simulink model "posture_reg_with_odoloc_Euler"  (Simulink 8.7)
settings: Solver=ode45  StartTime=0.0  StopTime=T  MaxStep=0.01  RelTol=1e-3
values from neighbouring files (symbols this model uses):
  T_s = 0.01    [init.m]
  theta_0 = pi/2    (= 1.57079632679)    [init.m]
  x_0 = -1    [init.m]
  y_0 = -2    [init.m]
undefined symbols (not defined in the file or in its folder): post_reg, wrap
settings Model: Creator=marilena  LastModifiedBy=giuseppe  ExtModeAutoUpdateStatusClock=off
settings DataIOCC: SignalLoggingSaveFormat=ModelDataLogs
settings OptimizationCC: ExpressionDepthLimit=2147483647
settings DebuggingCC: SaveWithParameterizedLinksMsg=none  SolverPrmCheckMsg=warning  FcnCallInpInsideContextMsg=UseLocalSettings  StateNameClashWarn=warning
settings HardwareCC: TargetHWDeviceType=32-bit Generic
settings GRTTargetCC: TargetFcnLib=ansi_tfl_tmw.mat  GeneratePreprocessorConditionals=Use local settings  CombineOutputUpdateFcns=off  GRTInterface=on

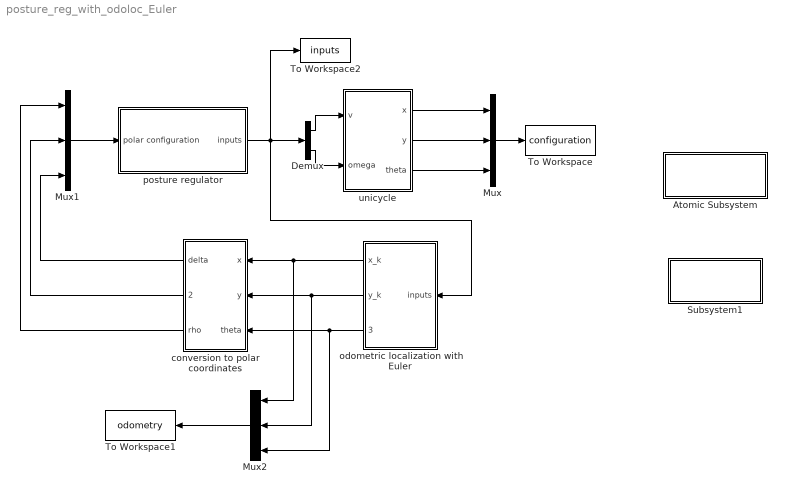
== system posture_reg_with_odoloc_Euler ==
  Atomic Subsystem : Subsystem  TreatAsAtomicUnit=on
      settings: OpenFcn=init
      mask Display: disp('initialization')
  Demux : Demux  Outputs=2
  Mux : Mux  Inputs=3
  Mux1 : Mux  Inputs=3
  Mux2 : Mux  Inputs=3
  Subsystem1 : Subsystem
      settings: OpenFcn=plots
      mask Display: disp('plots')
  To Workspace : ToWorkspace  VariableName=configuration  SaveFormat=Structure With Time
  To Workspace1 : ToWorkspace  VariableName=odometry  SaveFormat=Structure With Time
  To Workspace2 : ToWorkspace  VariableName=inputs  SaveFormat=Structure With Time
  conversion to polar coordinates : Subsystem
  odometric localization with Euler : Subsystem
  posture regulator : Subsystem
  unicycle : Subsystem
  wires:
  Mux/1 -> To Workspace/1
  unicycle/3(theta) -> Mux/3
  unicycle/1(x) -> Mux/1
  Mux1/1 -> posture regulator/1(polar configuration)
  posture regulator/1(inputs) -> odometric localization with Euler/1(inputs), Demux/1, To Workspace2/1
  unicycle/2(y) -> Mux/2
  Demux/1 -> unicycle/1(v)
  Demux/2 -> unicycle/2(omega)
  odometric localization with Euler/1(x_k) -> Mux2/1, conversion to polar coordinates/1(x)
  odometric localization with Euler/2(y_k) -> Mux2/2, conversion to polar coordinates/2(y)
  odometric localization with Euler/3(theta_k) -> Mux2/3, conversion to polar coordinates/3(theta)
  conversion to polar coordinates/1(delta) -> Mux1/3
  conversion to polar coordinates/2(gamma) -> Mux1/2
  conversion to polar coordinates/3(rho) -> Mux1/1
  Mux2/1 -> To Workspace1/1

== system posture_reg_with_odoloc_Euler/Atomic Subsystem ==

== system posture_reg_with_odoloc_Euler/Subsystem1 ==

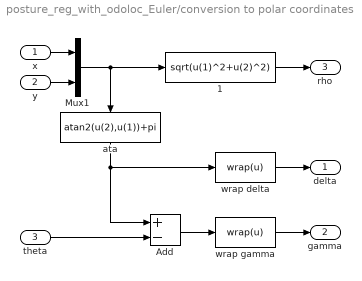
== system posture_reg_with_odoloc_Euler/conversion to polar coordinates ==
  x : Inport
  y : Inport  Port=2
  theta : Inport  Port=3
  " 1" : Fcn  Expr=sqrt(u(1)^2+u(2)^2)
  Add : Sum  Inputs=+-
  Mux1 : Mux  Inputs=2
  ata : Fcn  Expr=atan2(u(2),u(1))+pi
  wrap delta : MATLABFcn  MATLABFcn=wrap(u)
  wrap gamma : MATLABFcn  MATLABFcn=wrap(u)
  delta : Outport
  gamma : Outport  Port=2
  rho : Outport  Port=3
  wires:
  Mux1/1 -> " 1"/1, ata/1
  ata/1 -> Add/1, wrap delta/1
  x/1 -> Mux1/1
  " 1"/1 -> rho/1
  y/1 -> Mux1/2
  theta/1 -> Add/2
  wrap delta/1 -> delta/1
  Add/1 -> wrap gamma/1
  wrap gamma/1 -> gamma/1

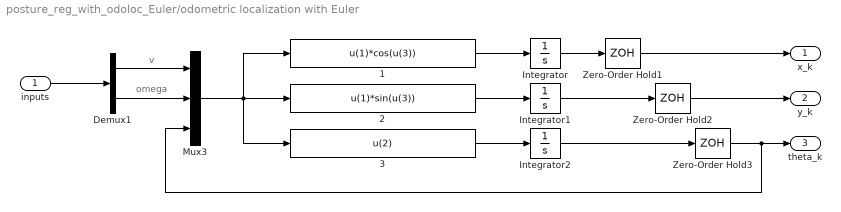
== system posture_reg_with_odoloc_Euler/odometric localization with Euler ==
  note: omega
  note: v
  inputs : Inport
  " 1" : Fcn  Expr=u(1)*cos(u(3))
  " 2" : Fcn  Expr=u(1)*sin(u(3))
  " 3" : Fcn  Expr=u(2)
  Demux1 : Demux  Outputs=2
  Integrator : Integrator  InitialCondition=x_0
  Integrator1 : Integrator  InitialCondition=y_0
  Integrator2 : Integrator  InitialCondition=theta_0
  Mux3 : Mux  Inputs=3
  Zero-Order Hold1 : ZeroOrderHold  SampleTime=T_s
  Zero-Order Hold2 : ZeroOrderHold  SampleTime=T_s
  Zero-Order Hold3 : ZeroOrderHold  SampleTime=T_s
  x_k : Outport
  y_k : Outport  Port=2
  theta_k : Outport  Port=3
  wires:
  " 1"/1 -> Integrator/1
  " 2"/1 -> Integrator1/1
  Mux3/1 -> " 3"/1, " 1"/1, " 2"/1
  " 3"/1 -> Integrator2/1
  Integrator/1 -> Zero-Order Hold1/1
  Integrator1/1 -> Zero-Order Hold2/1
  Integrator2/1 -> Zero-Order Hold3/1
  Zero-Order Hold3/1 -> Mux3/3, theta_k/1
  Zero-Order Hold2/1 -> y_k/1
  Zero-Order Hold1/1 -> x_k/1
  Demux1/1 -> Mux3/1
  Demux1/2 -> Mux3/2
  inputs/1 -> Demux1/1

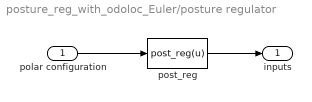
== system posture_reg_with_odoloc_Euler/posture regulator ==
  polar configuration : Inport
  post_reg : MATLABFcn  Tag={'prova'}  Description=cartesian regulator  MATLABFcn=post_reg(u)  Output1D=off
  inputs : Outport
  wires:
  polar configuration/1 -> post_reg/1
  post_reg/1 -> inputs/1

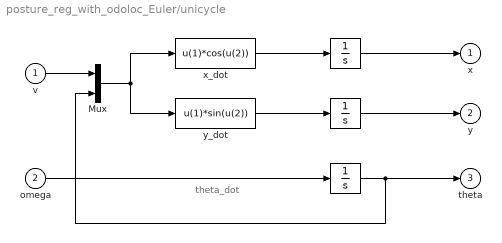
== system posture_reg_with_odoloc_Euler/unicycle ==
  note: theta_dot
  v : Inport
  omega : Inport  Port=2
  " " : Integrator  InitialCondition=theta_0
  "   " : Integrator  InitialCondition=x_0
  "    " : Integrator  InitialCondition=y_0
  Mux : Mux  Inputs=2
  x_dot : Fcn  Expr=u(1)*cos(u(2))
  y_dot : Fcn  Expr=u(1)*sin(u(2))
  x : Outport
  y : Outport  Port=2
  theta : Outport  Port=3
  wires:
  v/1 -> Mux/1
  omega/1 -> " "/1
  x_dot/1 -> "   "/1
  y_dot/1 -> "    "/1
  " "/1 -> Mux/2, theta/1
  Mux/1 -> x_dot/1, y_dot/1
  "   "/1 -> x/1
  "    "/1 -> y/1
